simulink model "vms_new_ut"  (Simulink 8.1)
settings: Solver=FixedStepDiscrete  StartTime=0.0  StopTime=10.0  FixedStep=0.005  RelTol=1e-3
libraries: siltestlib x6, vms_new x1
settings Model: Creator=xsellart  LastModifiedBy=AT015555
settings DataIOCC: SignalLoggingSaveFormat=Dataset
settings OptimizationCC: ExpressionDepthLimit=128
settings DebuggingCC: FcnCallInpInsideContextMsg=EnableAllAsError
settings GRTTargetCC: CombineOutputUpdateFcns=on  GRTInterface=off

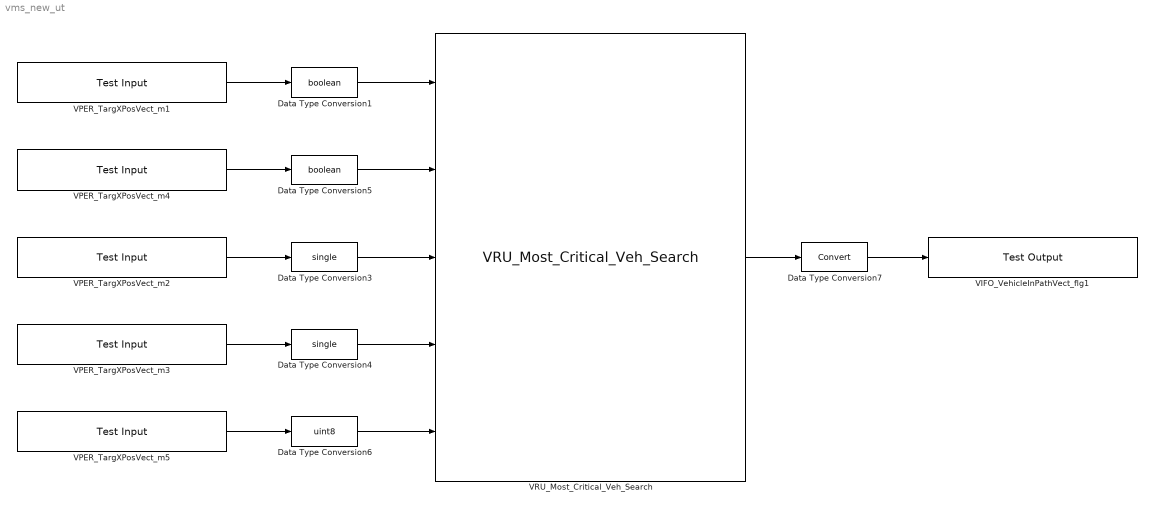
== system vms_new_ut ==
  Data Type Conversion1 : DataTypeConversion  OutDataTypeStr=boolean
  Data Type Conversion3 : DataTypeConversion  OutDataTypeStr=single
  Data Type Conversion4 : DataTypeConversion  OutDataTypeStr=single
  Data Type Conversion5 : DataTypeConversion  OutDataTypeStr=boolean
  Data Type Conversion6 : DataTypeConversion  OutDataTypeStr=uint8
  Data Type Conversion7 : DataTypeConversion
  VIFO_VehicleInPathVect_flg1 : siltestlib/Test Output  varname=VIFO_VRUMCTTargId_num  sampletime=-1
  VPER_TargXPosVect_m1 : siltestlib/Test Input  varname=NIFO_IsPotential_flg  sampletime=0.005
  VPER_TargXPosVect_m2 : siltestlib/Test Input  varname=VIFO_VRUSimpleTTCX_s  sampletime=0.005
  VPER_TargXPosVect_m3 : siltestlib/Test Input  varname=NIFO_VRUTargetNExistProb_num  sampletime=0.005
  VPER_TargXPosVect_m4 : siltestlib/Test Input  varname=VIFO_AEBTargetIsPed_flg  sampletime=0.005
  VPER_TargXPosVect_m5 : siltestlib/Test Input  varname=NIFO_IterationN_enum  sampletime=0.005
  VRU_Most_Critical_Veh_Search : vms_new/VRU_Most_Critical_Veh_Search
  wires:
  VPER_TargXPosVect_m1/1 -> Data Type Conversion1/1
  Data Type Conversion1/1 -> VRU_Most_Critical_Veh_Search/1
  VPER_TargXPosVect_m4/1 -> Data Type Conversion5/1
  Data Type Conversion5/1 -> VRU_Most_Critical_Veh_Search/2
  VPER_TargXPosVect_m2/1 -> Data Type Conversion3/1
  Data Type Conversion3/1 -> VRU_Most_Critical_Veh_Search/3
  VPER_TargXPosVect_m3/1 -> Data Type Conversion4/1
  Data Type Conversion4/1 -> VRU_Most_Critical_Veh_Search/4
  VPER_TargXPosVect_m5/1 -> Data Type Conversion6/1
  Data Type Conversion6/1 -> VRU_Most_Critical_Veh_Search/5
  Data Type Conversion7/1 -> VIFO_VehicleInPathVect_flg1/1
  VRU_Most_Critical_Veh_Search/1 -> Data Type Conversion7/1
